simulink model "sunsensor_processing_test"  (R2016b)
settings: Solver=VariableStepAuto  StartTime=0.0  StopTime=100  RelTol=1e-3
values from neighbouring files (symbols this model uses):
  fsw_params = init_fsw_params()    [sunsensor_processing_test_init.m]    (also in sunsensor_valid_flag_test_init.m)
libraries: GPS_time_lib x1, sun_sensor_lib x1, sun_vector_lib x1, sensor_processing_libs x1, time_coord_rotation_lib x1, tle2eci_coarse_lib x1
settings Model: Creator=Taylor  LastModifiedBy=Taylor

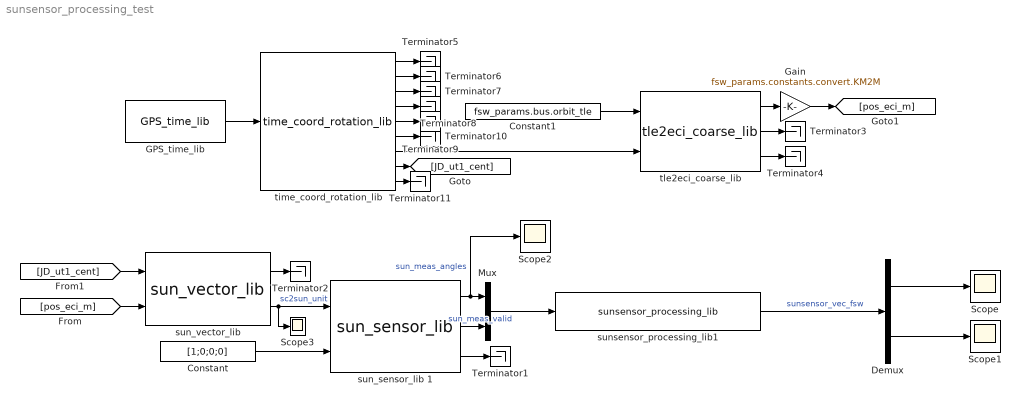
== system sunsensor_processing_test ==
  Constant : Constant  Value=[1;0;0;0]
  Constant1 : Constant  Value=fsw_params.bus.orbit_tle
  Demux : Demux  Outputs=[3 1]
  GPS_time_lib : GPS_time_lib/GPS_time_lib
  Gain : Gain  Gain=fsw_params.constants.convert.KM2M
  Mux : Mux  Inputs=[2 1]
  Scope{,1..3} (4 alike) : Scope
  Terminator{1..11} (11 alike) : Terminator
  sun_sensor_lib 1 : sun_sensor_lib/sun_sensor_lib 
  sun_vector_lib : sun_vector_lib/sun_vector_lib
  sunsensor_processing_lib1 : sensor_processing_libs/sunsensor_processing_lib
  time_coord_rotation_lib : time_coord_rotation_lib/time_coord_rotation_lib
  tle2eci_coarse_lib : tle2eci_coarse_lib/tle2eci_coarse_lib
  wires:
  sun_sensor_lib 1/1 -> Scope2/1, Mux/1  "sun_meas_angles"
  Mux/1 -> sunsensor_processing_lib1/1
  sunsensor_processing_lib1/1 -> Demux/1  "sunsensor_vec_fsw"
  sun_sensor_lib 1/2 -> Mux/2  "sun_meas_valid"
  sun_sensor_lib 1/3 -> Terminator1/1
  Demux/1 -> Scope/1
  Demux/2 -> Scope1/1
  GPS_time_lib/1 -> time_coord_rotation_lib/1
  sun_vector_lib/1 -> Terminator2/1
  Constant/1 -> sun_sensor_lib 1/2
  sun_vector_lib/2 -> Scope3/1, sun_sensor_lib 1/1  "sc2sun_unit"
  time_coord_rotation_lib/8 -> [JD_ut1_cent]
  [JD_ut1_cent] -> sun_vector_lib/1
  Constant1/1 -> tle2eci_coarse_lib/1
  tle2eci_coarse_lib/1 -> Gain/1
  tle2eci_coarse_lib/2 -> Terminator3/1
  Gain/1 -> [pos_eci_m]
  [pos_eci_m] -> sun_vector_lib/2
  time_coord_rotation_lib/7 -> tle2eci_coarse_lib/2
  tle2eci_coarse_lib/3 -> Terminator4/1
  time_coord_rotation_lib/1 -> Terminator5/1
  time_coord_rotation_lib/2 -> Terminator6/1
  time_coord_rotation_lib/3 -> Terminator7/1
  time_coord_rotation_lib/4 -> Terminator8/1
  time_coord_rotation_lib/5 -> Terminator9/1
  time_coord_rotation_lib/6 -> Terminator10/1
  time_coord_rotation_lib/9 -> Terminator11/1
